simulink model "RFC"  (R2019b)
settings: Solver=FixedStepDiscrete  StartTime=0  StopTime=5  FixedStep=fixedStepSize  MaxStep=0.001  RelTol=1e-3  EnableMultiTasking=on
model workspace (MAT data in the model file):
  Occurrence.FaultRemote = 1
  Occurrence.FaultLow = 2
  Occurrence.FaultLow_2 = 3
  Occurrence.FaultModerate = 4
  Occurrence.FaultModerate_2 = 5
  Occurrence.FaultModerate_3 = 6
  Occurrence.FaultHigh = 7
  Occurrence.FaultHigh_2 = 8
  Occurrence.Tolerance = 9
  Occurrence.OK = 10
  Partitions.Last = ''
  Partitions.All = '*'
  Severity.OK = 0
  Severity.Warn = 1
  Severity.VeryMinor = 2
  Severity.Minor = 3
  Severity.VeryLow = 4
  Severity.Low = 5
  Severity.Moderate = 6
  Severity.High = 7
  Severity.VeryHigh = 8
  Severity.HazardousWithWarning = 9
  Severity.HazardousNoWarning = 10
  Severity.Error = 11
  Severity.ErrorFatal = 20
  block : handle (value not decoded)
  t = 0
  time = 0
undefined symbols (not defined in the file): fixedStepSize, RFC_notAlwaysTime, RFC_preconditions_gear, RFC_preconditions_rpmLimit, RFC_preconditions_speedLimit, RFC_preconditions_throttleLimit, RFC_preconditions_torqueLimit, RFC_subsystem1_downThreshold1, RFC_subsystem1_downThreshold2, RFC_subsystem1_evChangesTime, RFC_subsystem1_evChangesTime2, RFC_subsystem1_gear, RFC_subsystem1_gearState, RFC_subsystem1_notAlwaysTime, RFC_subsystem1_rpmLimit, RFC_subsystem1_torqueLimit
libraries: simulink x4
settings Model: RequirementInfo={} %GIDa_2eec5742_b109_443f_bad2_42d52c6309f7  conn_id=-1  report_delay=1  Creator=aande176  LastModifiedBy=alex
settings SolverCC: AutoInsertRateTranBlk=on
settings DataIOCC: ExternalInput=[],CPSRSts__CPSRSts,[],[],[],[],[],[],[],LvTestSts__LvTestSts,IsgPwrLimMin__IsgPwrLimMin,[],IsgPwrLimMax__IsgPwrLimMax,TqAvlIntFromIfCpt__TqAvlIntFromIfCpt,[],[],[],[],[],TqAllwdInt__TqAllwdInt,[],[],[],[],[],[],[],HvBattUDynMaxLim__HvBattUDynMaxLim,[],HvBattUDynMinLim__HvBattUDynMinLim,[],InitCmpl__InitCmpl,[],[],[],[],[],[],[],[],[],[],[],HvTestSts__HvTestSts,[],[],[],IsgModReq__IsgModReq,[],[],[],[],[],[],[],[],[],[],[],[],[],[],[],[],[],EngSt1WdSts__EngSt1WdSts__IsUpdated,IsgSpdReq__IsgSpdReq__IsUpdated,IsgModReq__IsgModReq__IsUpdated,HvSysRlySts__HvSysRlySts__IsUpdated,HvSysRlySts_toController,[],[],[],[],ImobPrpsnAllwd__ImobPrpsnAllwd__dummy,[],[],[],[],ImobTurnOffAllwd__ImobTurnOffAllwd__dummy,[],[],[],No_GearEven,B_CloseClutchOdd,B_CloseClutchEven,[],[],[],B_EnableVSpAct,V_Vehicle_SetPoint_mps,[]  SaveFormat=StructureWithTime  SaveOutput=off  SaveTime=off  ReturnWorkspaceOutputs=off  SignalLoggingName=slunit_logdata
settings OptimizationCC: DefaultParameterBehavior=Inlined  ExpressionDepthLimit=2147483647  LifeSpan=Inf
settings DebuggingCC: RTPrefix=warning  AlgebraicLoopMsg=error  CheckSSInitialOutputMsg=off  SolverPrmCheckMsg=warning  IntegerOverflowMsg=none  ParameterPrecisionLossMsg=none  FcnCallInpInsideContextMsg=warning  BusObjectLabelMismatch=error  ModelReferenceDataLoggingMessage=none  StateNameClashWarn=warning  SFUnexpectedBacktrackingDiag=warning  SFNoUnconditionalDefaultTransitionDiag=warning  SFExecutionAtInitializationDiag=none  IntegerSaturationMsg=none  ArithmeticOperatorsInVariantConditions=warning
settings HardwareCC: ProdBitPerLong=64  ProdHWDeviceType=Intel->x86-64
settings ModelReferenceCC: UpdateModelReferenceTargets=AssumeUpToDate  PropagateSignalLabelsOutOfModel=off
settings SFSimCC: SimUseLocalCustomCode=off  SimGenImportedTypeDefs=on  CustomCodeUndefinedFunction=UseInterfaceOnly
settings RTWCC: RTWUseLocalCustomCode=off  RTWUseSimCustomCode=on
settings CodeAppCC: StateflowObjectComments=on
settings GRTTargetCC: TargetLangStandard=C89/C90 (ANSI)  GeneratePreprocessorConditionals=Disable all  CombineOutputUpdateFcns=off  MatFileLogging=off  GRTInterface=on
settings ConfigComp: CovScope=Subsystem  CovPath=RequirementsEvaluation/AvailableTorque  CovMetricSettings=dcw  CovHTMLOptions=-sRT=1 -aTS=1 -bRG=1 -bTC=1 -hTR=0 -nFC=0 -scm=1 -bcm=1 -xEv=0  CovHtmlReporting=on  CovSaveCumulativeToWorkspaceVar=on  CovSaveSingleToWorkspaceVar=on  CovExternalEMLEnable=off

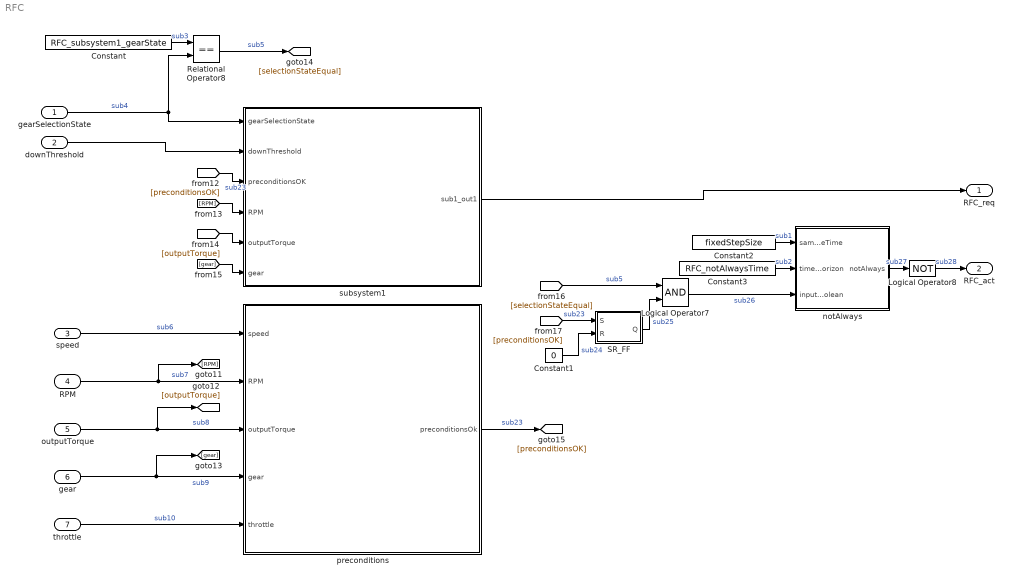
== system RFC ==
  gearSelectionState : Inport  PortDimensions=1  Interpolate=off
  downThreshold : Inport  Port=2  PortDimensions=1
  speed : Inport  Port=3  PortDimensions=1
  RPM : Inport  Port=4  PortDimensions=1
  outputTorque : Inport  Port=5  PortDimensions=1
  gear : Inport  Port=6
  throttle : Inport  Port=7  PortDimensions=1  Interpolate=off
  Constant : Constant  Value=RFC_subsystem1_gearState
  Constant1 : Constant  Value=0  OutDataTypeStr=boolean
  Constant2 : Constant  Value=fixedStepSize
  Constant3 : Constant  Value=RFC_notAlwaysTime
  Logical Operator7 : Logic  AllPortsSameDT=off  OutDataTypeStr=boolean
  Logical Operator8 : Logic  Operator=NOT  AllPortsSameDT=off  OutDataTypeStr=boolean
  Relational Operator8 : RelationalOperator  Operator===  OutDataTypeStr=boolean  RndMeth=Nearest
  SR_FF : Subsystem
      settings: CopyFcn=set_param(gcbh,'LinkStatus','none');
  notAlways : Subsystem
      settings: CopyFcn=set_param(gcbh,'LinkStatus','none');
  preconditions : Subsystem
  subsystem1 : Subsystem
  RFC_req : Outport  OutDataTypeStr=boolean  PortDimensions=1
  RFC_act : Outport  Port=2  OutDataTypeStr=boolean  PortDimensions=1
  wires:
  speed/1 -> preconditions/1(speed)  "sub6"
  Constant/1 -> Relational Operator8/1  "sub3"
  SR_FF/1(Q) -> Logical Operator7/2  "sub25"
  Constant1/1 -> SR_FF/2(R)  "sub24"
  [preconditionsOK] -> subsystem1/3(preconditionsOK)  "sub23"
  [preconditionsOK] -> SR_FF/1(S)  "sub23"
  Logical Operator7/1 -> notAlways/3(inputBoolean)  "sub26"
  [selectionStateEqual] -> Logical Operator7/1  "sub5"
  RPM/1 -> [RPM], preconditions/2(RPM)  "sub7"
  notAlways/1(notAlways) -> Logical Operator8/1  "sub27"
  preconditions/1(preconditionsOk) -> [preconditionsOK]  "sub23"
  throttle/1 -> preconditions/5(throttle)  "sub10"
  subsystem1/1(sub1_out1) -> RFC_req/1
  Relational Operator8/1 -> [selectionStateEqual]  "sub5"
  [RPM] -> subsystem1/4(RPM)
  gearSelectionState/1 -> Relational Operator8/2, subsystem1/1(gearSelectionState)  "sub4"
  [outputTorque] -> subsystem1/5(outputTorque)
  outputTorque/1 -> [outputTorque], preconditions/3(outputTorque)  "sub8"
  downThreshold/1 -> subsystem1/2(downThreshold)
  gear/1 -> [gear], preconditions/4(gear)  "sub9"
  Constant3/1 -> notAlways/2(timeHorizon)  "sub2"
  Constant2/1 -> notAlways/1(sampleTime)  "sub1"
  [gear] -> subsystem1/6(gear)
  Logical Operator8/1 -> RFC_act/1  "sub28"

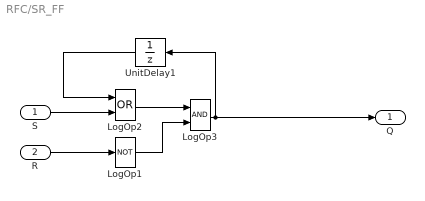
== system RFC/SR_FF ==
  S : Inport  OutDataTypeStr=boolean
  R : Inport  Port=2  OutDataTypeStr=boolean
  LogOp1 : Logic  Tag=struct('inputs','1','comment',struct('text','','placement',1),'logdata',struct('maxnumvals',4096,'plotchannels',[],'loggingmode',3,'channels',1),'operator','NOT','output',struct('class','default','description','','address','','unit','-','name','$S_$B','variable','','type','Bool'),'date',733638.68643228011,'scalingvalid',0)  Operator=NOT  Inputs=1  OutDataTypeStr=boolean
  LogOp2 : Logic  Tag=struct('inputs','2','comment',struct('text','','placement',1),'logdata',struct('maxnumvals',4096,'plotchannels',[],'loggingmode',3,'channels',1),'operator','AND','output',struct('class','default','description','','address','','unit','-','name','$S_$B','variable','','type','Bool'),'date',733638.68643680552,'scalingvalid',0)  Operator=OR  OutDataTypeStr=boolean
  LogOp3 : Logic  Tag=struct('inputs','2','comment',struct('text','','placement',1),'logdata',struct('maxnumvals',4096,'plotchannels',[],'loggingmode',3,'channels',1),'operator','OR','output',struct('class','default','description','','address','','unit','-','name','$S_$B','variable','','type','Bool'),'date',733638.68644151615,'scalingvalid',0)  OutDataTypeStr=boolean
  UnitDelay1 : UnitDelay  Tag=struct('comment',struct('text','','placement',1),'logdata',struct('maxnumvals',4096,'plotchannels',[],'loggingmode',3,'channels',1),'output',struct('width',1,'name','$S_$B','unit','','type','Bool','offset',0,'max',NaN,'min',NaN,'freeze',1,'lsb',1,'arb',0,'class','default','address','','description','','autoscalingmode',1,'lowerheadroom',1,'upperheadroom',1,'headroomunit','bit','checkmin',0,'checkmax',0,'show',0,'variable','','scaling','','keepdatatype',1,'castoutput',0),'state',struct('variable','','description','','name','X_$S_$B','width',1,'address','','max',NaN,'min',NaN,'class','default','type','Bool','scaling','','lsb',1,'offset',0,'arb',0,'freeze',1,'unit','','initial','0'),'dt','-1','date',733638.68644640048,'scalingvalid',0)  SampleTime=-1  HasFrameUpgradeWarning=on
  Q : Outport  OutDataTypeStr=boolean  VectorParamsAs1DForOutWhenUnconnected=off
  wires:
  UnitDelay1/1 -> LogOp2/1
  S/1 -> LogOp2/2
  R/1 -> LogOp1/1
  LogOp2/1 -> LogOp3/1
  LogOp1/1 -> LogOp3/2
  LogOp3/1 -> UnitDelay1/1, Q/1

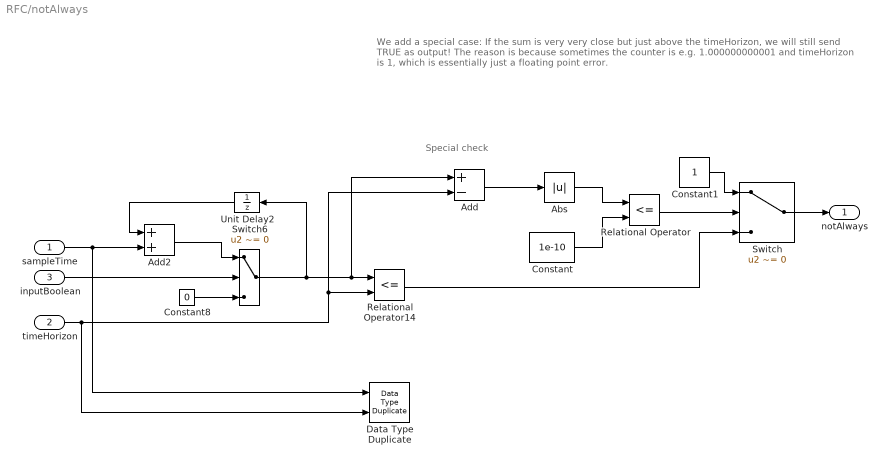
== system RFC/notAlways ==
  note: Special check
  note: We add a special case:
      | If the sum is very very close but just above the timeHorizon, we will still send TRUE as output!
      |
      | The reason is because sometimes the counter is e.g. 1.000000000001 and timeHorizon is 1, which is essentially just a floating point error.
  sampleTime : Inport
  timeHorizon : Inport  Port=2
  inputBoolean : Inport  Port=3
  Abs : Abs
  Add : Sum  Inputs=+-
  Add2 : Sum
  Constant : Constant  Value=1e-10
  Constant1 : Constant  OutDataTypeStr=boolean
  Constant8 : Constant  Value=0  OutDataTypeStr=Inherit: Inherit via back propagation
  Data Type Duplicate : DataTypeDuplicate
  Relational Operator : RelationalOperator  Operator=<=  OutDataTypeStr=boolean  RndMeth=Simplest
  Relational Operator14 : RelationalOperator  Operator=<=  OutDataTypeStr=boolean  RndMeth=Nearest
  Switch : Switch  Criteria=u2 ~= 0
  Switch6 : Switch  Criteria=u2 ~= 0
  Unit Delay2 : UnitDelay  SampleTime=-1  HasFrameUpgradeWarning=on
  notAlways : Outport  VectorParamsAs1DForOutWhenUnconnected=off
  wires:
  Switch6/1 -> Add/1, Relational Operator14/1, Unit Delay2/1
  timeHorizon/1 -> Add/2, Relational Operator14/2, Data Type Duplicate/2
  Relational Operator14/1 -> Switch/3
  Unit Delay2/1 -> Add2/1
  Add2/1 -> Switch6/1
  sampleTime/1 -> Add2/2, Data Type Duplicate/1
  Constant8/1 -> Switch6/3
  inputBoolean/1 -> Switch6/2
  Add/1 -> Abs/1
  Abs/1 -> Relational Operator/1
  Constant/1 -> Relational Operator/2
  Relational Operator/1 -> Switch/2
  Constant1/1 -> Switch/1
  Switch/1 -> notAlways/1

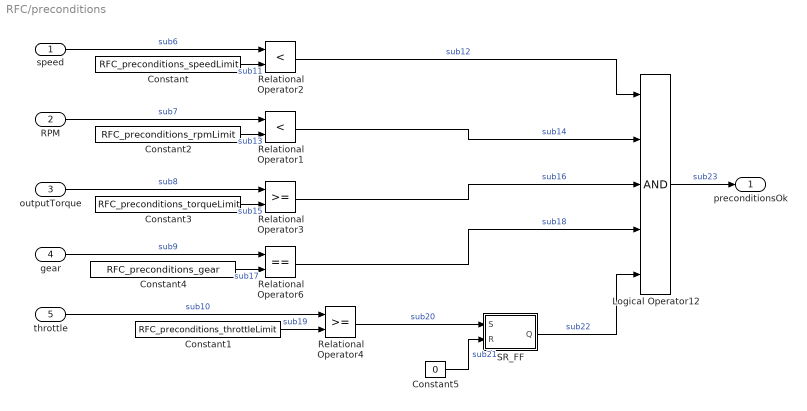
== system RFC/preconditions ==
  speed : Inport  PortDimensions=1
  RPM : Inport  Port=2
  outputTorque : Inport  Port=3
  gear : Inport  Port=4
  throttle : Inport  Port=5
  Constant : Constant  Value=RFC_preconditions_speedLimit
  Constant1 : Constant  Value=RFC_preconditions_throttleLimit
  Constant2 : Constant  Value=RFC_preconditions_rpmLimit
  Constant3 : Constant  Value=RFC_preconditions_torqueLimit
  Constant4 : Constant  Value=RFC_preconditions_gear
  Constant5 : Constant  Value=0  OutDataTypeStr=boolean
  Logical Operator12 : Logic  Inputs=5  AllPortsSameDT=off  OutDataTypeStr=boolean
  Relational Operator1 : RelationalOperator  Operator=<  OutDataTypeStr=boolean  RndMeth=Nearest
  Relational Operator2 : RelationalOperator  Operator=<  OutDataTypeStr=boolean  RndMeth=Nearest
  Relational Operator3 : RelationalOperator  OutDataTypeStr=boolean  RndMeth=Nearest
  Relational Operator4 : RelationalOperator  OutDataTypeStr=boolean  RndMeth=Nearest
  Relational Operator6 : RelationalOperator  Operator===  OutDataTypeStr=boolean  RndMeth=Nearest
  SR_FF : Subsystem
      settings: CopyFcn=set_param(gcbh,'LinkStatus','none');
  preconditionsOk : Outport
  wires:
  RPM/1 -> Relational Operator1/1  "sub7"
  Logical Operator12/1 -> preconditionsOk/1  "sub23"
  SR_FF/1(Q) -> Logical Operator12/5  "sub22"
  throttle/1 -> Relational Operator4/1  "sub10"
  outputTorque/1 -> Relational Operator3/1  "sub8"
  Constant3/1 -> Relational Operator3/2  "sub15"
  Relational Operator3/1 -> Logical Operator12/3  "sub16"
  Constant5/1 -> SR_FF/2(R)  "sub21"
  Constant/1 -> Relational Operator2/2  "sub11"
  Relational Operator2/1 -> Logical Operator12/1  "sub12"
  speed/1 -> Relational Operator2/1  "sub6"
  Relational Operator1/1 -> Logical Operator12/2  "sub14"
  Constant2/1 -> Relational Operator1/2  "sub13"
  gear/1 -> Relational Operator6/1  "sub9"
  Constant4/1 -> Relational Operator6/2  "sub17"
  Relational Operator6/1 -> Logical Operator12/4  "sub18"
  Constant1/1 -> Relational Operator4/2  "sub19"
  Relational Operator4/1 -> SR_FF/1(S)  "sub20"

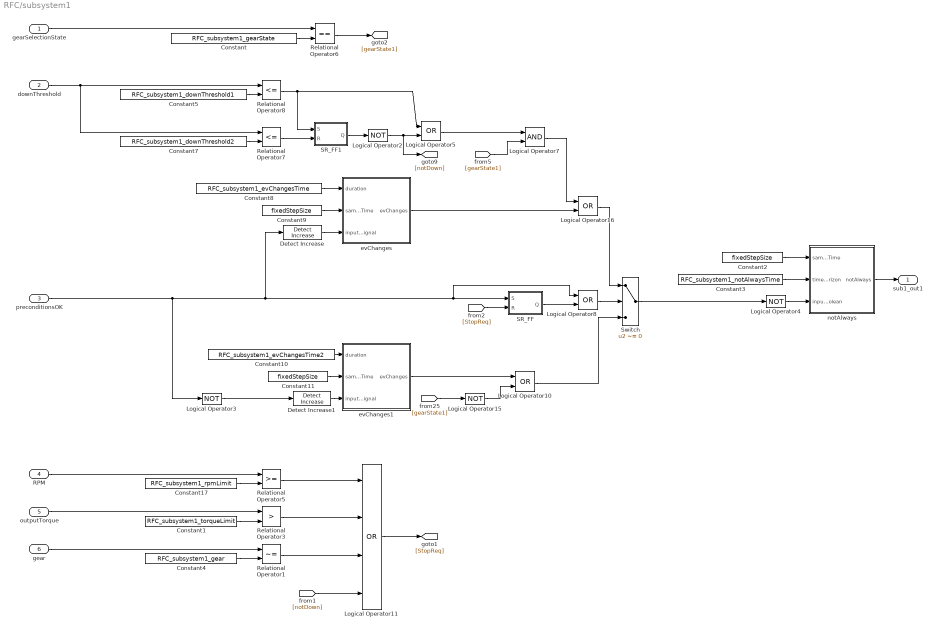
== system RFC/subsystem1 ==
  gearSelectionState : Inport
  downThreshold : Inport  Port=2
  preconditionsOK : Inport  Port=3
  RPM : Inport  Port=4
  outputTorque : Inport  Port=5
  gear : Inport  Port=6
  Constant : Constant  Value=RFC_subsystem1_gearState
  Constant1 : Constant  Value=RFC_subsystem1_torqueLimit
  Constant10 : Constant  Value=RFC_subsystem1_evChangesTime2
  Constant11 : Constant  Value=fixedStepSize
  Constant17 : Constant  Value=RFC_subsystem1_rpmLimit
  Constant2 : Constant  Value=fixedStepSize
  Constant3 : Constant  Value=RFC_subsystem1_notAlwaysTime
  Constant4 : Constant  Value=RFC_subsystem1_gear
  Constant5 : Constant  Value=RFC_subsystem1_downThreshold1
  Constant7 : Constant  Value=RFC_subsystem1_downThreshold2
  Constant8 : Constant  Value=RFC_subsystem1_evChangesTime
  Constant9 : Constant  Value=fixedStepSize
  Detect Increase : simulink/Logic and Bit Operations/Detect Increase  vinit=0  OutDataTypeStr=boolean
  Detect Increase1 : simulink/Logic and Bit Operations/Detect Increase  vinit=0  OutDataTypeStr=boolean
  Logical Operator{5,8,10,16} (4 alike) : Logic  Operator=OR  AllPortsSameDT=off  OutDataTypeStr=boolean
  Logical Operator11 : Logic  Operator=OR  Inputs=4  AllPortsSameDT=off  OutDataTypeStr=boolean
  Logical Operator{2..4,15} (4 alike) : Logic  Operator=NOT  AllPortsSameDT=off  OutDataTypeStr=boolean
  Logical Operator7 : Logic  AllPortsSameDT=off  OutDataTypeStr=boolean
  Relational Operator1 : RelationalOperator  Operator=~=  OutDataTypeStr=boolean  RndMeth=Nearest
  Relational Operator3 : RelationalOperator  Operator=>  OutDataTypeStr=boolean  RndMeth=Nearest
  Relational Operator5 : RelationalOperator  OutDataTypeStr=boolean  RndMeth=Nearest
  Relational Operator6 : RelationalOperator  Operator===  OutDataTypeStr=boolean  RndMeth=Nearest
  Relational Operator7 : RelationalOperator  Operator=<=  OutDataTypeStr=boolean  RndMeth=Nearest
  Relational Operator8 : RelationalOperator  Operator=<=  OutDataTypeStr=boolean  RndMeth=Nearest
  SR_FF : Subsystem
      settings: CopyFcn=set_param(gcbh,'LinkStatus','none');
  SR_FF1 : Subsystem
      settings: CopyFcn=set_param(gcbh,'LinkStatus','none');
  Switch : Switch  Criteria=u2 ~= 0
  evChanges : Subsystem
      settings: CopyFcn=set_param(gcbh,'LinkStatus','none');
  evChanges1 : Subsystem
      settings: CopyFcn=set_param(gcbh,'LinkStatus','none');
  notAlways : Subsystem
      settings: CopyFcn=set_param(gcbh,'LinkStatus','none');
  sub1_out1 : Outport
  wires:
  Logical Operator5/1 -> Logical Operator7/1
  preconditionsOK/1 -> SR_FF/1(S), Logical Operator8/1, Detect Increase/1, Logical Operator3/1
  notAlways/1(notAlways) -> sub1_out1/1
  Constant3/1 -> notAlways/2(timeHorizon)
  Constant2/1 -> notAlways/1(sampleTime)
  Logical Operator4/1 -> notAlways/3(inputBoolean)
  Relational Operator7/1 -> SR_FF1/2(R)
  Constant10/1 -> evChanges1/1(duration)
  Constant11/1 -> evChanges1/2(sampleTime)
  Switch/1 -> Logical Operator4/1
  Logical Operator16/1 -> Switch/1
  [gearState1] -> Logical Operator7/2
  evChanges1/1(evChanges) -> Logical Operator10/1
  Logical Operator10/1 -> Switch/3
  [gearState1] -> Logical Operator15/1
  Logical Operator15/1 -> Logical Operator10/2
  evChanges/1(evChanges) -> Logical Operator16/2
  Constant9/1 -> evChanges/2(sampleTime)
  Constant8/1 -> evChanges/1(duration)
  Logical Operator2/1 -> [notDown], Logical Operator5/2
  SR_FF1/1(Q) -> Logical Operator2/1
  gearSelectionState/1 -> Relational Operator6/1
  Constant/1 -> Relational Operator6/2
  Relational Operator6/1 -> [gearState1]
  downThreshold/1 -> Relational Operator8/1, Relational Operator7/1
  Constant7/1 -> Relational Operator7/2
  Constant5/1 -> Relational Operator8/2
  Relational Operator8/1 -> SR_FF1/1(S), Logical Operator5/1
  Logical Operator7/1 -> Logical Operator16/1
  SR_FF/1(Q) -> Logical Operator8/2
  [StopReq] -> SR_FF/2(R)
  Detect Increase/1 -> evChanges/3(inputSignal)
  Logical Operator8/1 -> Switch/2
  Logical Operator3/1 -> Detect Increase1/1
  Detect Increase1/1 -> evChanges1/3(inputSignal)
  RPM/1 -> Relational Operator5/1
  Constant17/1 -> Relational Operator5/2
  outputTorque/1 -> Relational Operator3/1
  Constant1/1 -> Relational Operator3/2
  gear/1 -> Relational Operator1/1
  Constant4/1 -> Relational Operator1/2
  Relational Operator3/1 -> Logical Operator11/2
  Relational Operator1/1 -> Logical Operator11/3
  Relational Operator5/1 -> Logical Operator11/1
  [notDown] -> Logical Operator11/4
  Logical Operator11/1 -> [StopReq]

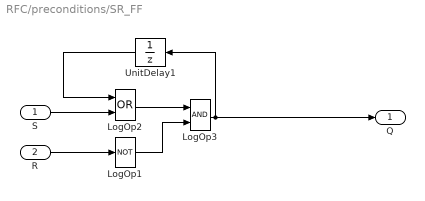
== system RFC/preconditions/SR_FF ==
  S : Inport  OutDataTypeStr=boolean
  R : Inport  Port=2  OutDataTypeStr=boolean
  LogOp1 : Logic  Tag=struct('inputs','1','comment',struct('text','','placement',1),'logdata',struct('maxnumvals',4096,'plotchannels',[],'loggingmode',3,'channels',1),'operator','NOT','output',struct('class','default','description','','address','','unit','-','name','$S_$B','variable','','type','Bool'),'date',733638.68643228011,'scalingvalid',0)  Operator=NOT  Inputs=1  OutDataTypeStr=boolean
  LogOp2 : Logic  Tag=struct('inputs','2','comment',struct('text','','placement',1),'logdata',struct('maxnumvals',4096,'plotchannels',[],'loggingmode',3,'channels',1),'operator','AND','output',struct('class','default','description','','address','','unit','-','name','$S_$B','variable','','type','Bool'),'date',733638.68643680552,'scalingvalid',0)  Operator=OR  OutDataTypeStr=boolean
  LogOp3 : Logic  Tag=struct('inputs','2','comment',struct('text','','placement',1),'logdata',struct('maxnumvals',4096,'plotchannels',[],'loggingmode',3,'channels',1),'operator','OR','output',struct('class','default','description','','address','','unit','-','name','$S_$B','variable','','type','Bool'),'date',733638.68644151615,'scalingvalid',0)  OutDataTypeStr=boolean
  UnitDelay1 : UnitDelay  Tag=struct('comment',struct('text','','placement',1),'logdata',struct('maxnumvals',4096,'plotchannels',[],'loggingmode',3,'channels',1),'output',struct('width',1,'name','$S_$B','unit','','type','Bool','offset',0,'max',NaN,'min',NaN,'freeze',1,'lsb',1,'arb',0,'class','default','address','','description','','autoscalingmode',1,'lowerheadroom',1,'upperheadroom',1,'headroomunit','bit','checkmin',0,'checkmax',0,'show',0,'variable','','scaling','','keepdatatype',1,'castoutput',0),'state',struct('variable','','description','','name','X_$S_$B','width',1,'address','','max',NaN,'min',NaN,'class','default','type','Bool','scaling','','lsb',1,'offset',0,'arb',0,'freeze',1,'unit','','initial','0'),'dt','-1','date',733638.68644640048,'scalingvalid',0)  SampleTime=-1  HasFrameUpgradeWarning=on
  Q : Outport  OutDataTypeStr=boolean  VectorParamsAs1DForOutWhenUnconnected=off
  wires:
  UnitDelay1/1 -> LogOp2/1
  S/1 -> LogOp2/2
  R/1 -> LogOp1/1
  LogOp2/1 -> LogOp3/1
  LogOp1/1 -> LogOp3/2
  LogOp3/1 -> UnitDelay1/1, Q/1

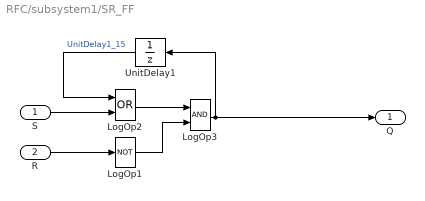
== system RFC/subsystem1/SR_FF ==
  S : Inport  OutDataTypeStr=boolean
  R : Inport  Port=2  OutDataTypeStr=boolean
  LogOp1 : Logic  Tag=struct('inputs','1','comment',struct('text','','placement',1),'logdata',struct('maxnumvals',4096,'plotchannels',[],'loggingmode',3,'channels',1),'operator','NOT','output',struct('class','default','description','','address','','unit','-','name','$S_$B','variable','','type','Bool'),'date',733638.68643228011,'scalingvalid',0)  Operator=NOT  Inputs=1  OutDataTypeStr=boolean
  LogOp2 : Logic  Tag=struct('inputs','2','comment',struct('text','','placement',1),'logdata',struct('maxnumvals',4096,'plotchannels',[],'loggingmode',3,'channels',1),'operator','AND','output',struct('class','default','description','','address','','unit','-','name','$S_$B','variable','','type','Bool'),'date',733638.68643680552,'scalingvalid',0)  Operator=OR  OutDataTypeStr=boolean
  LogOp3 : Logic  Tag=struct('inputs','2','comment',struct('text','','placement',1),'logdata',struct('maxnumvals',4096,'plotchannels',[],'loggingmode',3,'channels',1),'operator','OR','output',struct('class','default','description','','address','','unit','-','name','$S_$B','variable','','type','Bool'),'date',733638.68644151615,'scalingvalid',0)  OutDataTypeStr=boolean
  UnitDelay1 : UnitDelay  Tag=struct('comment',struct('text','','placement',1),'logdata',struct('maxnumvals',4096,'plotchannels',[],'loggingmode',3,'channels',1),'output',struct('width',1,'name','$S_$B','unit','','type','Bool','offset',0,'max',NaN,'min',NaN,'freeze',1,'lsb',1,'arb',0,'class','default','address','','description','','autoscalingmode',1,'lowerheadroom',1,'upperheadroom',1,'headroomunit','bit','checkmin',0,'checkmax',0,'show',0,'variable','','scaling','','keepdatatype',1,'castoutput',0),'state',struct('variable','','description','','name','X_$S_$B','width',1,'address','','max',NaN,'min',NaN,'class','default','type','Bool','scaling','','lsb',1,'offset',0,'arb',0,'freeze',1,'unit','','initial','0'),'dt','-1','date',733638.68644640048,'scalingvalid',0)  SampleTime=-1  HasFrameUpgradeWarning=on
  Q : Outport  OutDataTypeStr=boolean  VectorParamsAs1DForOutWhenUnconnected=off
  wires:
  UnitDelay1/1 -> LogOp2/1  "UnitDelay1_15"
  S/1 -> LogOp2/2
  R/1 -> LogOp1/1
  LogOp2/1 -> LogOp3/1
  LogOp1/1 -> LogOp3/2
  LogOp3/1 -> UnitDelay1/1, Q/1

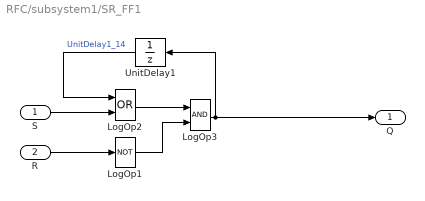
== system RFC/subsystem1/SR_FF1 ==
  S : Inport  OutDataTypeStr=boolean
  R : Inport  Port=2  OutDataTypeStr=boolean
  LogOp1 : Logic  Tag=struct('inputs','1','comment',struct('text','','placement',1),'logdata',struct('maxnumvals',4096,'plotchannels',[],'loggingmode',3,'channels',1),'operator','NOT','output',struct('class','default','description','','address','','unit','-','name','$S_$B','variable','','type','Bool'),'date',733638.68643228011,'scalingvalid',0)  Operator=NOT  Inputs=1  OutDataTypeStr=boolean
  LogOp2 : Logic  Tag=struct('inputs','2','comment',struct('text','','placement',1),'logdata',struct('maxnumvals',4096,'plotchannels',[],'loggingmode',3,'channels',1),'operator','AND','output',struct('class','default','description','','address','','unit','-','name','$S_$B','variable','','type','Bool'),'date',733638.68643680552,'scalingvalid',0)  Operator=OR  OutDataTypeStr=boolean
  LogOp3 : Logic  Tag=struct('inputs','2','comment',struct('text','','placement',1),'logdata',struct('maxnumvals',4096,'plotchannels',[],'loggingmode',3,'channels',1),'operator','OR','output',struct('class','default','description','','address','','unit','-','name','$S_$B','variable','','type','Bool'),'date',733638.68644151615,'scalingvalid',0)  OutDataTypeStr=boolean
  UnitDelay1 : UnitDelay  Tag=struct('comment',struct('text','','placement',1),'logdata',struct('maxnumvals',4096,'plotchannels',[],'loggingmode',3,'channels',1),'output',struct('width',1,'name','$S_$B','unit','','type','Bool','offset',0,'max',NaN,'min',NaN,'freeze',1,'lsb',1,'arb',0,'class','default','address','','description','','autoscalingmode',1,'lowerheadroom',1,'upperheadroom',1,'headroomunit','bit','checkmin',0,'checkmax',0,'show',0,'variable','','scaling','','keepdatatype',1,'castoutput',0),'state',struct('variable','','description','','name','X_$S_$B','width',1,'address','','max',NaN,'min',NaN,'class','default','type','Bool','scaling','','lsb',1,'offset',0,'arb',0,'freeze',1,'unit','','initial','0'),'dt','-1','date',733638.68644640048,'scalingvalid',0)  SampleTime=-1  HasFrameUpgradeWarning=on
  Q : Outport  OutDataTypeStr=boolean  VectorParamsAs1DForOutWhenUnconnected=off
  wires:
  UnitDelay1/1 -> LogOp2/1  "UnitDelay1_14"
  S/1 -> LogOp2/2
  R/1 -> LogOp1/1
  LogOp2/1 -> LogOp3/1
  LogOp1/1 -> LogOp3/2
  LogOp3/1 -> UnitDelay1/1, Q/1

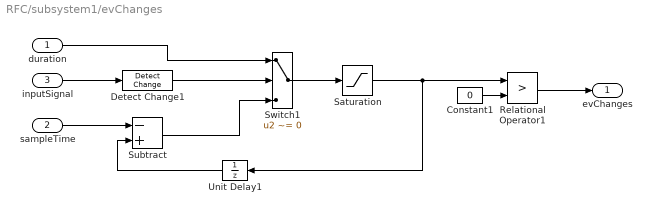
== system RFC/subsystem1/evChanges ==
  duration : Inport
  sampleTime : Inport  Port=2
  inputSignal : Inport  Port=3
  Constant1 : Constant  Value=0
  Detect Change1 : simulink/Logic and Bit Operations/Detect Change  vinit=0  OutDataTypeStr=boolean
  Relational Operator1 : RelationalOperator  Operator=>  OutDataTypeStr=boolean  RndMeth=Nearest
  Saturation : Saturate  UpperLimit=Inf  LowerLimit=0
  Subtract : Sum  Inputs=-+
  Switch1 : Switch  Criteria=u2 ~= 0
  Unit Delay1 : UnitDelay  SampleTime=-1  HasFrameUpgradeWarning=on
  evChanges : Outport  VectorParamsAs1DForOutWhenUnconnected=off
  wires:
  Detect Change1/1 -> Switch1/2
  duration/1 -> Switch1/1
  Switch1/1 -> Saturation/1
  inputSignal/1 -> Detect Change1/1
  Constant1/1 -> Relational Operator1/2
  Subtract/1 -> Switch1/3
  Saturation/1 -> Relational Operator1/1, Unit Delay1/1
  Unit Delay1/1 -> Subtract/2
  Relational Operator1/1 -> evChanges/1
  sampleTime/1 -> Subtract/1

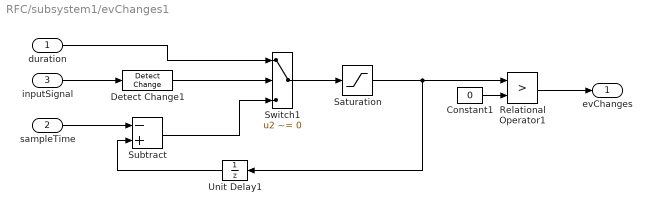
== system RFC/subsystem1/evChanges1 ==
  duration : Inport
  sampleTime : Inport  Port=2
  inputSignal : Inport  Port=3
  Constant1 : Constant  Value=0
  Detect Change1 : simulink/Logic and Bit Operations/Detect Change  vinit=0  OutDataTypeStr=boolean
  Relational Operator1 : RelationalOperator  Operator=>  OutDataTypeStr=boolean  RndMeth=Nearest
  Saturation : Saturate  UpperLimit=Inf  LowerLimit=0
  Subtract : Sum  Inputs=-+
  Switch1 : Switch  Criteria=u2 ~= 0
  Unit Delay1 : UnitDelay  SampleTime=-1  HasFrameUpgradeWarning=on
  evChanges : Outport  VectorParamsAs1DForOutWhenUnconnected=off
  wires:
  Detect Change1/1 -> Switch1/2
  duration/1 -> Switch1/1
  Switch1/1 -> Saturation/1
  inputSignal/1 -> Detect Change1/1
  Constant1/1 -> Relational Operator1/2
  Subtract/1 -> Switch1/3
  Saturation/1 -> Relational Operator1/1, Unit Delay1/1
  Unit Delay1/1 -> Subtract/2
  Relational Operator1/1 -> evChanges/1
  sampleTime/1 -> Subtract/1

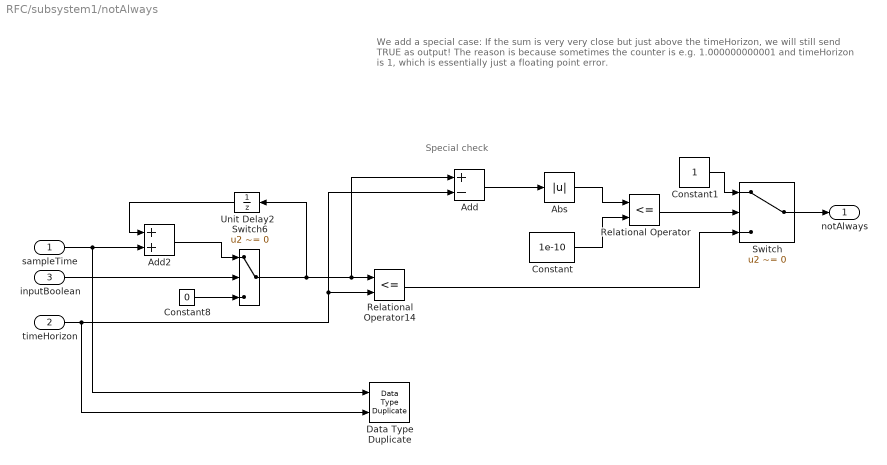
== system RFC/subsystem1/notAlways ==
  note: Special check
  note: We add a special case:
      | If the sum is very very close but just above the timeHorizon, we will still send TRUE as output!
      |
      | The reason is because sometimes the counter is e.g. 1.000000000001 and timeHorizon is 1, which is essentially just a floating point error.
  sampleTime : Inport
  timeHorizon : Inport  Port=2
  inputBoolean : Inport  Port=3
  Abs : Abs
  Add : Sum  Inputs=+-
  Add2 : Sum
  Constant : Constant  Value=1e-10
  Constant1 : Constant  OutDataTypeStr=boolean
  Constant8 : Constant  Value=0  OutDataTypeStr=Inherit: Inherit via back propagation
  Data Type Duplicate : DataTypeDuplicate
  Relational Operator : RelationalOperator  Operator=<=  OutDataTypeStr=boolean  RndMeth=Simplest
  Relational Operator14 : RelationalOperator  Operator=<=  OutDataTypeStr=boolean  RndMeth=Nearest
  Switch : Switch  Criteria=u2 ~= 0
  Switch6 : Switch  Criteria=u2 ~= 0
  Unit Delay2 : UnitDelay  SampleTime=-1  HasFrameUpgradeWarning=on
  notAlways : Outport  VectorParamsAs1DForOutWhenUnconnected=off
  wires:
  Switch6/1 -> Add/1, Relational Operator14/1, Unit Delay2/1
  timeHorizon/1 -> Add/2, Relational Operator14/2, Data Type Duplicate/2
  Relational Operator14/1 -> Switch/3
  Unit Delay2/1 -> Add2/1
  Add2/1 -> Switch6/1
  sampleTime/1 -> Add2/2, Data Type Duplicate/1
  Constant8/1 -> Switch6/3
  inputBoolean/1 -> Switch6/2
  Add/1 -> Abs/1
  Abs/1 -> Relational Operator/1
  Constant/1 -> Relational Operator/2
  Relational Operator/1 -> Switch/2
  Constant1/1 -> Switch/1
  Switch/1 -> notAlways/1
